simulink model "fourtank_OpenloopModel"  (R2024b)
settings: Solver=ode45  StartTime=0.0  StopTime=1800  MaxStep=5  MinStep=4  RelTol=1e-6  AbsTol=1e-6  EnableMultiTasking=on
InitFcn:
  | A1=28; A3=28;
  | A2=32; A4=32;
  | a1=0.071; a3=0.071;
  | a2=0.057; a4=0.057;
  | g=981;
settings Model: Creator=Anjali
settings SolverCC: InitialStep=4  ZeroCrossAlgorithm=Adaptive
settings DataIOCC: LimitDataPoints=on  SaveFormat=Array  SignalLoggingSaveFormat=ModelDataLogs  ReturnWorkspaceOutputs=off  SignalLoggingName=sigsOut  OutputOption=SpecifiedOutputTimes  OutputTimes=[0:1:1800]
settings OptimizationCC: BooleanDataType=off
settings DebuggingCC: SaveWithParameterizedLinksMsg=none  MergeDetectMultiDrivingBlocksExec=none  SignalResolutionControl=TryResolveAllWithWarning  MultiTaskDSMMsg=warning  MultiTaskCondExecSysMsg=none  UnconnectedInputMsg=warning  UnconnectedOutputMsg=warning  UnconnectedLineMsg=warning
settings HardwareCC: ProdBitPerPointer=32  ProdBitPerSizeT=32  ProdBitPerPtrDiffT=32  ProdLargestAtomicFloat=None  ProdIntDivRoundTo=Undefined  ProdEndianess=Unspecified  ProdWordSize=32  ProdHWDeviceType=32-bit Generic  TargetUnknown=on
settings ModelReferenceCC: PropagateSignalLabelsOutOfModel=off
settings GRTTargetCC: CombineOutputUpdateFcns=off  GRTInterface=on
settings ConfigComp: CovMetricSettings=dw  CovSaveCumulativeToWorkspaceVar=on  CovSaveSingleToWorkspaceVar=on

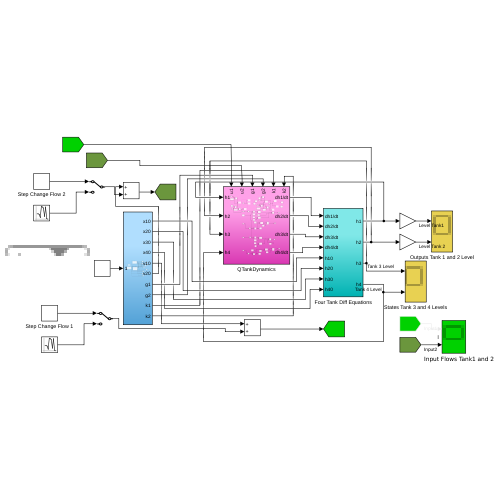
[thumbnail: Simulink's stored preview of the top-level diagram]
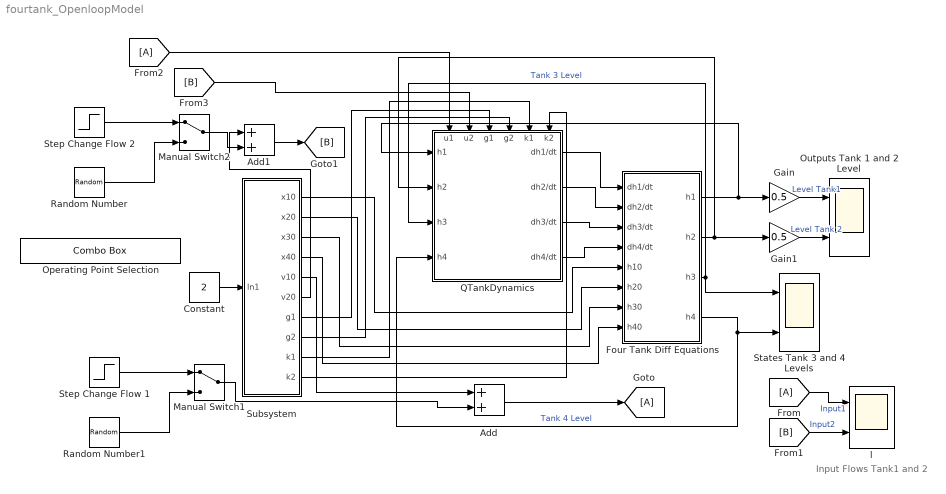
== system fourtank_OpenloopModel ==
  note: Input Flows Tank1 and 2
  Add : Sum
  Add1 : Sum
  Constant : Constant  Value=2
  Four Tank Diff Equations : Subsystem
  From : From
  From2 : From
  Gain : Gain  Gain=0.5  SaturateOnIntegerOverflow=on  OutDataTypeStr=Inherit: Same as input  ParamDataTypeStr=Inherit: Same as input
  Gain1 : Gain  Gain=0.5  SaturateOnIntegerOverflow=on  OutDataTypeStr=Inherit: Same as input  ParamDataTypeStr=Inherit: Same as input
  Goto : Goto
  Manual Switch1 : ManualSwitch
  Manual Switch2 : ManualSwitch
  Operating Point Selection : ComboBox  LabelPosition=Hide  SelectedLabel=Non-Minimum Phase
      settings: Values={{'Minimum Phase', 'Non-Minimum Phase'}, [1 2]}
  Outputs Tank 1 and 2 Level : Scope  NumInputPorts=2
  QTankDynamics : Subsystem
      settings: PortSchema="{\"entries\":[{\"content\":{\"sides\":[{\"content\":{\"connectorIds\":[\"In1\",\"In2\",\"In3\",\"In4\"]},\"type\":\"ConnectorPlacement.EquallySpacedRectSide\",\"uuid\":\"3a80b6b7-73e5-4221-8773-90f6774224f4\"},{\"content\":{\"connectorIds\":[\"Out1\",\"Out2\",\"Out3\",\"Out4\"],\"side\":\"RIGHT\"},\"type\":\"ConnectorPlacement.EquallySpacedRectSide\",\"uuid\":\"8dbf4ce3-8b66-4623-9c03-b1a8293bbc94\"},{\"content\":{\"connectorIds\":[\"In5\",\"In6\",\"In7\",\"In8\",\"In9\",\"In10\"],\"side\":\"TOP\"},\"type\":\"ConnectorPlacement.EquallySpacedRectSide\",\"uuid\":\"b8bae85a-0d15-4c72-a0c9-aef1eabdd2c9\"}]},\"type\":\"ConnectorPlacement.EquallySpacedConnector\",\"uuid\":\"356cf736-14a2-452f-9f0a-77a2cf0d6009\"}],\"packageUris\":[\"http://schema.mathworks.com/mf0/Connector/R2020b\"],\"version\":\"1.0\"}"
  Random Number : RandomNumber  SampleTime=6
  Random Number1 : RandomNumber  Variance=0.001  SampleTime=6
  States Tank 3 and 4 Levels : Scope  NumInputPorts=2
  Step Change Flow 1 : Step  Time=900  After=0.5  SampleTime=6
  Step Change Flow 2 : Step  Time=900  After=-0.5  SampleTime=6
  Subsystem : Subsystem
  l : Scope  NumInputPorts=2
  wires:
  Step Change Flow 1/1 -> Manual Switch1/1
  Subsystem/7(g1) -> QTankDynamics/7(g1)
  Step Change Flow 2/1 -> Manual Switch2/1
  [B] -> QTankDynamics/6(u2)
  Random Number/1 -> Manual Switch2/2
  From/1 -> l/1  "Input1"
  Constant/1 -> Subsystem/1(In1)
  Subsystem/2(x20) -> Four Tank Diff Equations/6(h20)
  Random Number1/1 -> Manual Switch1/2
  Four Tank Diff Equations/1(h1) -> Gain/1, QTankDynamics/1(h1)
  QTankDynamics/1(dh1/dt) -> Four Tank Diff Equations/1(dh1/dt)
  [B] -> l/2  "Input2"
  Four Tank Diff Equations/4(h4) -> QTankDynamics/4(h4), States Tank 3 and 4 Levels/2  "Tank 4 Level"
  From2/1 -> QTankDynamics/5(u1)
  Subsystem/1(x10) -> Four Tank Diff Equations/5(h10)
  Subsystem/3(x30) -> Four Tank Diff Equations/7(h30)
  Subsystem/4(x40) -> Four Tank Diff Equations/8(h40)
  Subsystem/5(v10) -> Add/1
  Subsystem/8(g2) -> QTankDynamics/8(g2)
  Manual Switch1/1 -> Add/2
  Subsystem/9(k1) -> QTankDynamics/9(k1)
  Subsystem/10(k2) -> QTankDynamics/10(k2)
  Add/1 -> Goto/1
  Add1/1 -> [B]
  QTankDynamics/2(dh2/dt) -> Four Tank Diff Equations/2(dh2/dt)
  QTankDynamics/3(dh3/dt) -> Four Tank Diff Equations/3(dh3/dt)
  QTankDynamics/4(dh4/dt) -> Four Tank Diff Equations/4(dh4/dt)
  Four Tank Diff Equations/2(h2) -> Gain1/1, QTankDynamics/2(h2)
  Four Tank Diff Equations/3(h3) -> States Tank 3 and 4 Levels/1, QTankDynamics/3(h3)  "Tank 3 Level"
  Gain/1 -> Outputs Tank 1 and 2 Level/1  "Level Tank1"
  Gain1/1 -> Outputs Tank 1 and 2 Level/2  "Level Tank 2"
  Manual Switch2/1 -> Add1/2
  Subsystem/6(v20) -> Add1/1

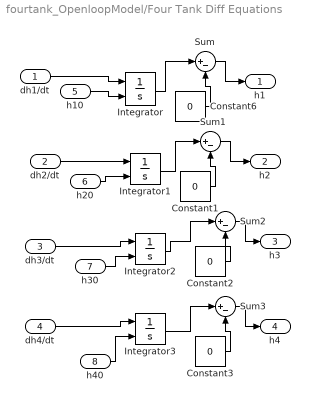
== system fourtank_OpenloopModel/Four Tank Diff Equations ==
  dh1/dt : Inport
  dh2/dt : Inport  Port=2
  dh3/dt : Inport  Port=3
  dh4/dt : Inport  Port=4
  h10 : Inport  Port=5
  h20 : Inport  Port=6
  h30 : Inport  Port=7
  h40 : Inport  Port=8
  Constant{1..3,6} (4 alike) : Constant  Value=0
  Integrator{,1..3} (4 alike) : Integrator  InitialConditionSource=external
  Sum{,1..3} (4 alike) : Sum  Inputs=|+-  SaturateOnIntegerOverflow=on
  h1 : Outport
  h2 : Outport  Port=2
  h3 : Outport  Port=3
  h4 : Outport  Port=4
  wires:
  dh1/dt/1 -> Integrator/1
  dh2/dt/1 -> Integrator1/1
  dh3/dt/1 -> Integrator2/1
  dh4/dt/1 -> Integrator3/1
  Integrator/1 -> Sum/1
  Constant6/1 -> Sum/2
  Sum/1 -> h1/1
  Integrator1/1 -> Sum1/1
  Constant1/1 -> Sum1/2
  Sum1/1 -> h2/1
  Integrator2/1 -> Sum2/1
  Constant2/1 -> Sum2/2
  Sum2/1 -> h3/1
  Integrator3/1 -> Sum3/1
  Constant3/1 -> Sum3/2
  Sum3/1 -> h4/1
  h20/1 -> Integrator1/2
  h30/1 -> Integrator2/2
  h40/1 -> Integrator3/2
  h10/1 -> Integrator/2

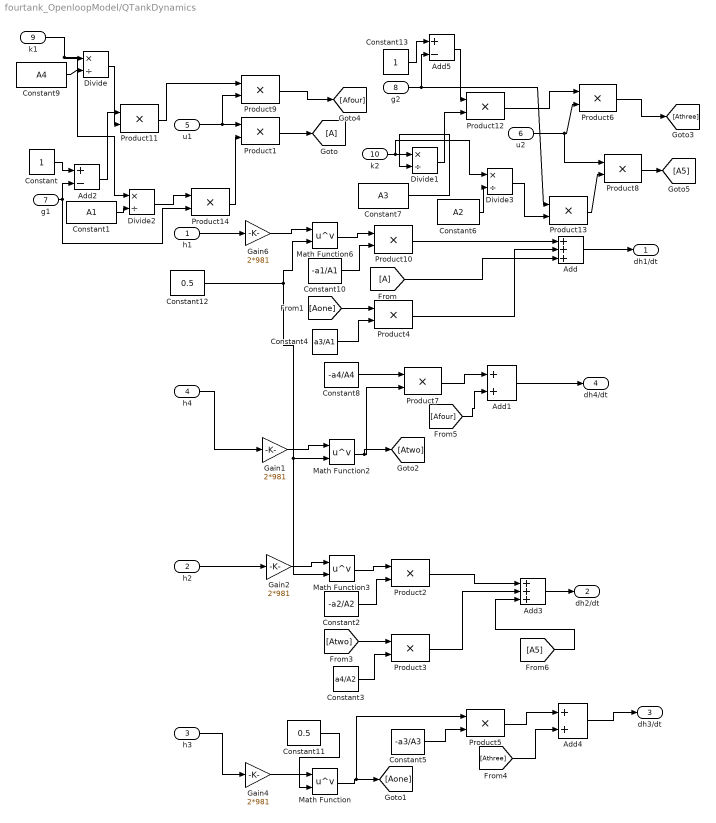
== system fourtank_OpenloopModel/QTankDynamics ==
  h1 : Inport
  h2 : Inport  Port=2
  h3 : Inport  Port=3
  h4 : Inport  Port=4
  u1 : Inport  Port=5
  u2 : Inport  Port=6
  g1 : Inport  Port=7
  g2 : Inport  Port=8
  k1 : Inport  Port=9
  k2 : Inport  Port=10
  Add : Sum  Inputs=+++
  Add1 : Sum
  Add2 : Sum  Inputs=+-
  Add3 : Sum  Inputs=+++
  Add4 : Sum
  Add5 : Sum  Inputs=+-
  Constant : Constant
  Constant1 : Constant  Value=A1
  Constant10 : Constant  Value=-a1/A1
  Constant11 : Constant  Value=0.5
  Constant12 : Constant  Value=0.5
  Constant13 : Constant
  Constant2 : Constant  Value=-a2/A2
  Constant3 : Constant  Value=a4/A2
  Constant4 : Constant  Value=a3/A1
  Constant5 : Constant  Value=-a3/A3
  Constant6 : Constant  Value=A2
  Constant7 : Constant  Value=A3
  Constant8 : Constant  Value=-a4/A4
  Constant9 : Constant  Value=A4
  Divide{,1..3} (4 alike) : Product  Inputs=*/
  From : From
  Gain{1..2,4,6} (4 alike) : Gain  Gain=2*981  SaturateOnIntegerOverflow=on  OutDataTypeStr=Inherit: Same as input  ParamDataTypeStr=Inherit: Same as input
  Goto : Goto
  Math Function : Math  Operator=pow
  Math Function2 : Math  Operator=pow  SignedPower=on
  Math Function3 : Math  Operator=pow  SignedPower=on
  Math Function6 : Math  Operator=pow  SignedPower=on
  Product{1..14} (14 alike) : Product  InputSameDT=on  SaturateOnIntegerOverflow=on  OutDataTypeStr=Inherit: Same as first input
  dh1/dt : Outport
  dh2/dt : Outport  Port=2
  dh3/dt : Outport  Port=3
  dh4/dt : Outport  Port=4
  wires:
  Add3/1 -> dh2/dt/1
  Product8/1 -> [A5]
  Constant8/1 -> Product7/1
  Product4/1 -> Add/2
  Math Function6/1 -> Product10/1
  Constant4/1 -> Product4/2
  [Aone] -> Product4/1
  h4/1 -> Gain1/1
  h3/1 -> Gain4/1
  Gain6/1 -> Math Function6/1
  Constant10/1 -> Product10/2
  Product6/1 -> [Athree]
  Add1/1 -> dh4/dt/1
  Add/1 -> dh1/dt/1
  h2/1 -> Gain2/1
  u2/1 -> Product8/1, Product6/2
  Constant11/1 -> Math Function/2
  Math Function/1 -> Product5/1, [Aone]
  Math Function2/1 -> Product7/2, [Atwo]
  Constant2/1 -> Product2/2
  h1/1 -> Gain6/1
  Gain1/1 -> Math Function2/1
  Math Function3/1 -> Product2/1
  Constant3/1 -> Product3/2
  Product9/1 -> [Afour]
  Product1/1 -> Goto/1
  Add4/1 -> dh3/dt/1
  [Atwo] -> Product3/1
  Gain2/1 -> Math Function3/1
  Product3/1 -> Add3/2
  Product7/1 -> Add1/1
  [Athree] -> Add4/2
  Constant5/1 -> Product5/2
  Product5/1 -> Add4/1
  Constant12/1 -> Math Function6/2, Math Function3/2, Math Function2/2
  Product2/1 -> Add3/1
  Product10/1 -> Add/1
  [Afour] -> Add1/2
  Gain4/1 -> Math Function/1
  u1/1 -> Product9/2, Product1/1
  From/1 -> Add/3
  [A5] -> Add3/3
  Constant/1 -> Add2/1
  g1/1 -> Add2/2, Product14/2
  Add2/1 -> Product11/1
  Product11/1 -> Product9/1
  Constant13/1 -> Add5/1
  g2/1 -> Product13/1, Add5/2
  Add5/1 -> Product12/1
  Product12/1 -> Product6/1
  Constant9/1 -> Divide/2
  Divide/1 -> Product11/2
  k1/1 -> Divide2/1, Divide/1
  k2/1 -> Divide3/1, Divide1/1
  Constant7/1 -> Divide1/2
  Divide1/1 -> Product12/2
  Constant1/1 -> Divide2/2
  Divide2/1 -> Product14/1
  Product14/1 -> Product1/2
  Constant6/1 -> Divide3/2
  Divide3/1 -> Product13/2
  Product13/1 -> Product8/2

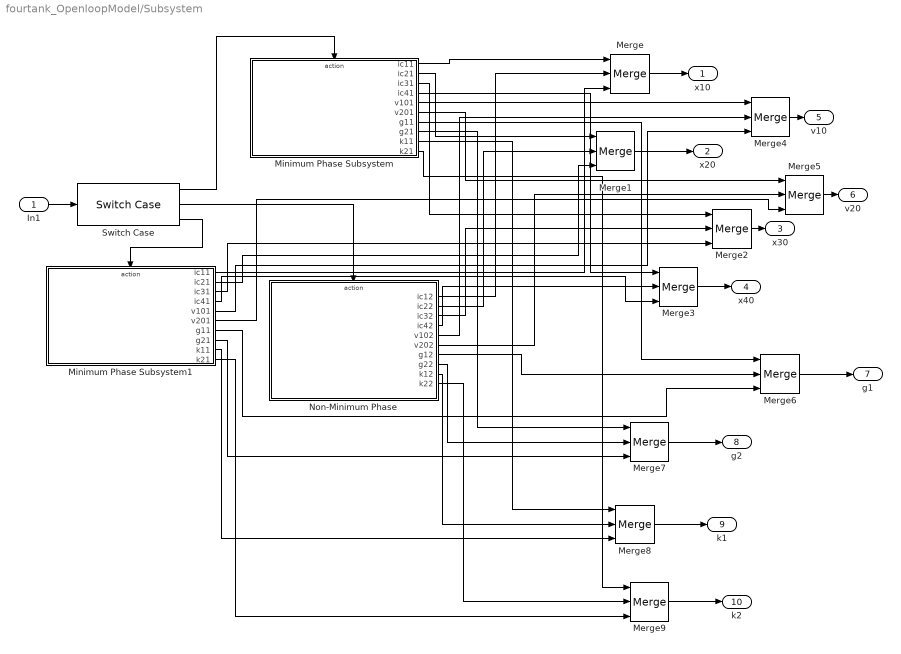
== system fourtank_OpenloopModel/Subsystem ==
  In1 : Inport
  Merge{,1..9} (10 alike) : Merge  Inputs=3
  Minimum Phase Subsystem : Subsystem  TreatAsAtomicUnit=on
  Minimum Phase Subsystem1 : Subsystem  TreatAsAtomicUnit=on
  Non-Minimum Phase : Subsystem  TreatAsAtomicUnit=on
  Switch Case : SwitchCase  CaseConditions={1 2}
  x10 : Outport
  x20 : Outport  Port=2
  x30 : Outport  Port=3
  x40 : Outport  Port=4
  v10 : Outport  Port=5
  v20 : Outport  Port=6
  g1 : Outport  Port=7
  g2 : Outport  Port=8
  k1 : Outport  Port=9
  k2 : Outport  Port=10
  wires:
  In1/1 -> Switch Case/1
  Switch Case/1 -> Minimum Phase Subsystem/Action
  Switch Case/2 -> Non-Minimum Phase/Action
  Minimum Phase Subsystem/4(ic41) -> Merge3/1
  Minimum Phase Subsystem/1(ic11) -> Merge/1
  Non-Minimum Phase/1(ic12) -> Merge/2
  Merge/1 -> x10/1
  Minimum Phase Subsystem/2(ic21) -> Merge1/1
  Merge1/1 -> x20/1
  Minimum Phase Subsystem/3(ic31) -> Merge2/1
  Non-Minimum Phase/3(ic32) -> Merge2/2
  Merge2/1 -> x30/1
  Non-Minimum Phase/4(ic42) -> Merge3/2
  Merge3/1 -> x40/1
  Non-Minimum Phase/2(ic22) -> Merge1/2
  Minimum Phase Subsystem/5(v101) -> Merge4/1
  Merge4/1 -> v10/1
  Non-Minimum Phase/5(v102) -> Merge4/2
  Minimum Phase Subsystem/6(v201) -> Merge5/1
  Non-Minimum Phase/6(v202) -> Merge5/2
  Merge5/1 -> v20/1
  Minimum Phase Subsystem/7(g11) -> Merge6/1
  Non-Minimum Phase/7(g12) -> Merge6/2
  Merge6/1 -> g1/1
  Merge7/1 -> g2/1
  Merge8/1 -> k1/1
  Merge9/1 -> k2/1
  Minimum Phase Subsystem/10(k21) -> Merge9/1
  Non-Minimum Phase/10(k22) -> Merge9/2
  Minimum Phase Subsystem/8(g21) -> Merge7/1
  Non-Minimum Phase/8(g22) -> Merge7/2
  Non-Minimum Phase/9(k12) -> Merge8/2
  Minimum Phase Subsystem/9(k11) -> Merge8/1
  Switch Case/3 -> Minimum Phase Subsystem1/Action
  Minimum Phase Subsystem1/1(ic11) -> Merge/3
  Minimum Phase Subsystem1/2(ic21) -> Merge1/3
  Minimum Phase Subsystem1/3(ic31) -> Merge2/3
  Minimum Phase Subsystem1/4(ic41) -> Merge3/3
  Minimum Phase Subsystem1/5(v101) -> Merge4/3
  Minimum Phase Subsystem1/6(v201) -> Merge5/3
  Minimum Phase Subsystem1/7(g11) -> Merge6/3
  Minimum Phase Subsystem1/8(g21) -> Merge7/3
  Minimum Phase Subsystem1/9(k11) -> Merge8/3
  Minimum Phase Subsystem1/10(k21) -> Merge9/3

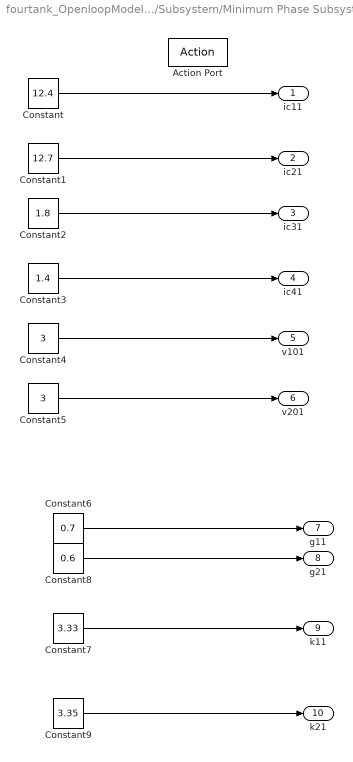
== system fourtank_OpenloopModel/Subsystem/Minimum Phase Subsystem ==
  Action Port : ActionPort  ActionPortLabel=case [ 1 ]:
  Constant : Constant  Value=12.4
  Constant1 : Constant  Value=12.7
  Constant2 : Constant  Value=1.8
  Constant3 : Constant  Value=1.4
  Constant4 : Constant  Value=3
  Constant5 : Constant  Value=3
  Constant6 : Constant  Value=0.7
  Constant7 : Constant  Value=3.33
  Constant8 : Constant  Value=0.6
  Constant9 : Constant  Value=3.35
  ic11 : Outport
  ic21 : Outport  Port=2
  ic31 : Outport  Port=3
  ic41 : Outport  Port=4
  v101 : Outport  Port=5
  v201 : Outport  Port=6
  g11 : Outport  Port=7
  g21 : Outport  Port=8
  k11 : Outport  Port=9
  k21 : Outport  Port=10
  wires:
  Constant3/1 -> ic41/1
  Constant/1 -> ic11/1
  Constant1/1 -> ic21/1
  Constant2/1 -> ic31/1
  Constant4/1 -> v101/1
  Constant5/1 -> v201/1
  Constant9/1 -> k21/1
  Constant6/1 -> g11/1
  Constant8/1 -> g21/1
  Constant7/1 -> k11/1

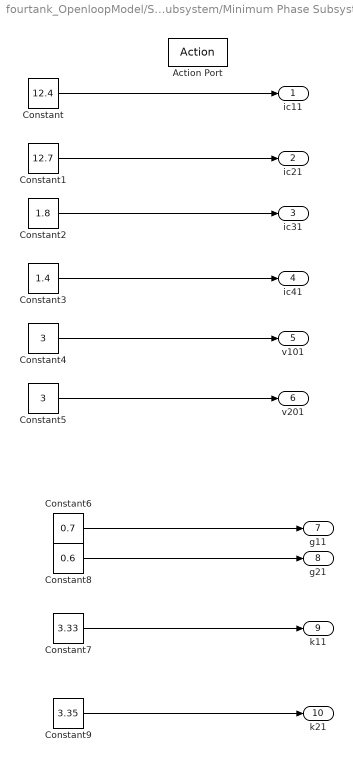
== system fourtank_OpenloopModel/Subsystem/Minimum Phase Subsystem1 ==
  Action Port : ActionPort  ActionPortLabel=default:
  Constant : Constant  Value=12.4
  Constant1 : Constant  Value=12.7
  Constant2 : Constant  Value=1.8
  Constant3 : Constant  Value=1.4
  Constant4 : Constant  Value=3
  Constant5 : Constant  Value=3
  Constant6 : Constant  Value=0.7
  Constant7 : Constant  Value=3.33
  Constant8 : Constant  Value=0.6
  Constant9 : Constant  Value=3.35
  ic11 : Outport
  ic21 : Outport  Port=2
  ic31 : Outport  Port=3
  ic41 : Outport  Port=4
  v101 : Outport  Port=5
  v201 : Outport  Port=6
  g11 : Outport  Port=7
  g21 : Outport  Port=8
  k11 : Outport  Port=9
  k21 : Outport  Port=10
  wires:
  Constant3/1 -> ic41/1
  Constant/1 -> ic11/1
  Constant1/1 -> ic21/1
  Constant2/1 -> ic31/1
  Constant4/1 -> v101/1
  Constant5/1 -> v201/1
  Constant9/1 -> k21/1
  Constant6/1 -> g11/1
  Constant8/1 -> g21/1
  Constant7/1 -> k11/1

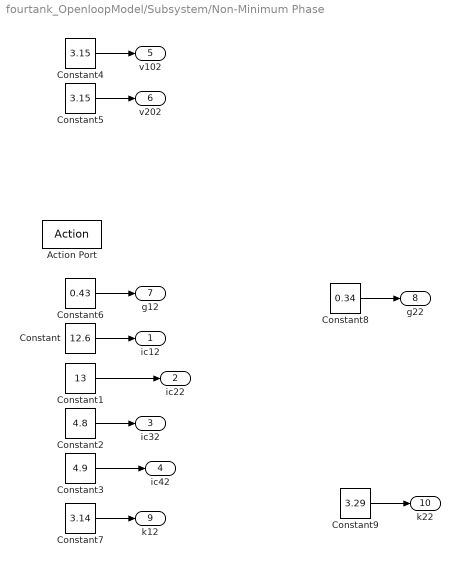
== system fourtank_OpenloopModel/Subsystem/Non-Minimum Phase ==
  Action Port : ActionPort  ActionPortLabel=case [ 2 ]:
  Constant : Constant  Value=12.6
  Constant1 : Constant  Value=13
  Constant2 : Constant  Value=4.8
  Constant3 : Constant  Value=4.9
  Constant4 : Constant  Value=3.15
  Constant5 : Constant  Value=3.15
  Constant6 : Constant  Value=0.43
  Constant7 : Constant  Value=3.14
  Constant8 : Constant  Value=0.34
  Constant9 : Constant  Value=3.29
  ic12 : Outport
  ic22 : Outport  Port=2
  ic32 : Outport  Port=3
  ic42 : Outport  Port=4
  v102 : Outport  Port=5
  v202 : Outport  Port=6
  g12 : Outport  Port=7
  g22 : Outport  Port=8
  k12 : Outport  Port=9
  k22 : Outport  Port=10
  wires:
  Constant3/1 -> ic42/1
  Constant2/1 -> ic32/1
  Constant4/1 -> v102/1
  Constant/1 -> ic12/1
  Constant1/1 -> ic22/1
  Constant5/1 -> v202/1
  Constant6/1 -> g12/1
  Constant9/1 -> k22/1
  Constant8/1 -> g22/1
  Constant7/1 -> k12/1
